simulink model "setModelStateTurtlebotROS"  (R2018a)
settings: Solver=FixedStepAuto  StartTime=0.0  StopTime=inf  FixedStep=0.1  RelTol=1e-3
model workspace (MAT data in the model file):
  SL_ROS_VariableLengthArrays_MaxSizes.CommonInfo.ArrayTruncateAction = 'EmitWarning'
  SL_ROS_VariableLengthArrays_MaxSizes.MsgTypeMap = containers.Map
  SL_ROS_VariableLengthArrays_MaxSizes.MsgTypeMap.serialization.keys = {'gazebo_msgs/ModelState'}
  SL_ROS_VariableLengthArrays_MaxSizes.MsgTypeMap.serialization.values{1}(1).PropertyName = 'ModelName'
  SL_ROS_VariableLengthArrays_MaxSizes.MsgTypeMap.serialization.values{1}(1).DataType = 'uint8'
  SL_ROS_VariableLengthArrays_MaxSizes.MsgTypeMap.serialization.values{1}(1).MaxLength = 11
  SL_ROS_VariableLengthArrays_MaxSizes.MsgTypeMap.serialization.values{1}(2).PropertyName = 'ReferenceFrame'
  SL_ROS_VariableLengthArrays_MaxSizes.MsgTypeMap.serialization.values{1}(2).DataType = 'uint8'
  SL_ROS_VariableLengthArrays_MaxSizes.MsgTypeMap.serialization.values{1}(2).MaxLength = 128
  SL_ROS_VariableLengthArrays_MaxSizes.MsgTypeMap.serialization.uniformity = 0
  SL_ROS_VariableLengthArrays_MaxSizes.MsgTypeMap.serialization.keyType = 'char'
  SL_ROS_VariableLengthArrays_MaxSizes.MsgTypeMap.serialization.valueType = 'any'
undefined symbols (not defined in the file): ModelName, ModelName_SL_Info, Pose
libraries: simulink x6, robotlib x2, sharedtransform x1
settings Model: EnablePacing=on  Creator=David  LastModifiedBy=David

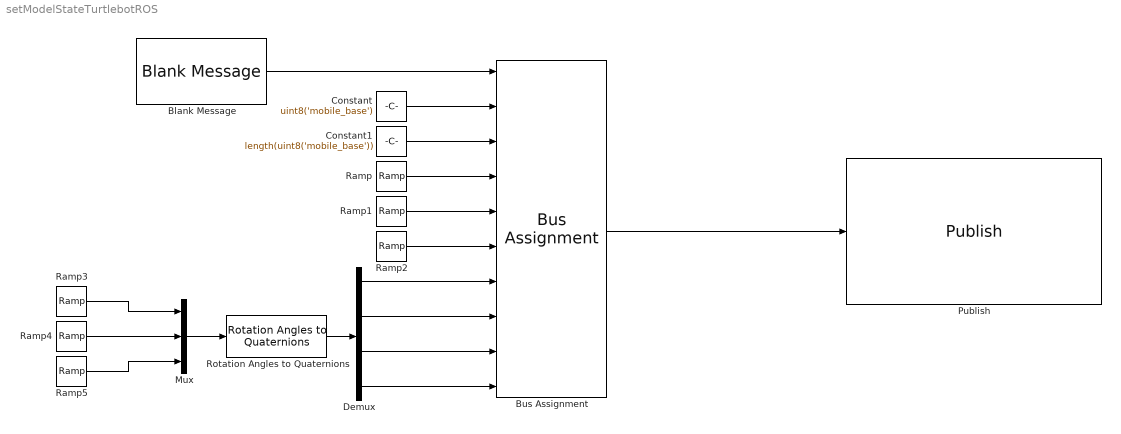
== system setModelStateTurtlebotROS ==
  Blank Message : robotlib/Blank Message  SourceLibraryInfo=This block requires Robotics System Toolbox  messageType=gazebo_msgs/ModelState  SampleTime=inf
      settings: SourceProductBaseCode=RO
  Bus Assignment : BusAssignment  AssignedSignals=ModelName,ModelName_SL_Info.CurrentLength,Pose.Position.X,Pose.Position.Y,Pose.Position.Z,Pose.Orientation.X,Pose.Orientation.Y,Pose.Orientation.Z,Pose.Orientation.W
  Constant : Constant  Value=uint8('mobile_base')
  Constant1 : Constant  Value=length(uint8('mobile_base'))  OutDataTypeStr=uint32
  Demux : Demux
  Mux : Mux  Inputs=3
  Publish : robotlib/Publish  SourceLibraryInfo=This block requires Robotics System Toolbox  topicSource=Select from ROS network  topic=/gazebo/set_model_state  messageType=gazebo_msgs/ModelState  messageQueueLength=1
      settings: SourceProductBaseCode=RO
  Ramp : simulink/Sources/Ramp  slope=0.1  start=2  InitialOutput=0
  Ramp1 : simulink/Sources/Ramp  slope=0.05  start=2  InitialOutput=0
  Ramp2 : simulink/Sources/Ramp  slope=0  start=2  InitialOutput=0
  Ramp3 : simulink/Sources/Ramp  slope=0  start=2  InitialOutput=pi
  Ramp4 : simulink/Sources/Ramp  slope=0  start=2  InitialOutput=0
  Ramp5 : simulink/Sources/Ramp  slope=10*pi/180  start=2  InitialOutput=0
  Rotation Angles to Quaternions : sharedtransform/Rotation Angles to Quaternions  rotationOrder=ZYX  aMode=aMode
      settings: SourceProductName=Aerospace Blockset  SourceProductBaseCode=AE
  wires:
  Blank Message/1 -> Bus Assignment/1
  Bus Assignment/1 -> Publish/1
  Ramp/1 -> Bus Assignment/4
  Ramp1/1 -> Bus Assignment/5
  Ramp2/1 -> Bus Assignment/6
  Constant/1 -> Bus Assignment/2
  Constant1/1 -> Bus Assignment/3
  Ramp3/1 -> Mux/1
  Ramp4/1 -> Mux/2
  Ramp5/1 -> Mux/3
  Mux/1 -> Rotation Angles to Quaternions/1
  Rotation Angles to Quaternions/1 -> Demux/1
  Demux/1 -> Bus Assignment/7
  Demux/2 -> Bus Assignment/8
  Demux/3 -> Bus Assignment/9
  Demux/4 -> Bus Assignment/10
